simulink library "trw_checksum"  (Simulink 8.2)
settings: Solver=ode1  StartTime=0.0  StopTime=Inf  FixedStep=0.001  RelTol=1e-3
PostLoadFcn:
  | , if any(exist('dsrtsu_mdlpostloadfcn', 'file') == [2, 3, 6]), try dsrtsu_mdlpostloadfcn('Execute', bdroot); catch fprintf('Error in PostLoadFcn (dsrtsu_mdlpostloadfcn) for model "%s":\n %s\n', bdroot, lasterr); end, end,
settings Model: DSRTSU_INTERNAL_RTI_VER=450  DSRTSU_INTERNAL_RTI_TYPE=rti1401  RTICANMMDATA=struct('GeneralSetupData',struct('modelroot','D:\ADAS\ADAS\trunk\ADAS_Softwares\HTDragon\software\sw_development\arch','generalsettings',struct('filesettings',struct('destfolder',struct('Name','RTICANMM_FILES','Check',1),'buildfolder',struct('Name','.','Check',1),'AbsDestfolder',struct('Name','D:\ADAS\ADAS\trunk\ADAS_Softwares\HTDragon\software\sw_development\arch\RTICANMM_FILES'),'AbsBuildfolder',struct('Name','D:\ADAS\ADAS\trunk\ADAS_Softwares\HTDragon\software\sw_development\arch'))),'options',struct('addpaths',1,'rmpaths',1,'addtrcexclusion',logical(1),'cannavigator',struct('checkmonitoring',0),'show_usrtrc',0,'use_usrtrc',0),'advanced',struct('options',[1 1 1 1 1 1 1 1 1 1 1 1 1 1 1 1 1 1 1 1 1 1 1 1 1 1 1 1 1 1 1 1 1 1 1 1 1 1 1 1 1 1 1 1 1 1 1 1 1 1 1 1 1 1 1 1 1 1 1 1 1 1 1 1 1 1 1 1 1 1 1 1 1 1 1 1 1 1 1 1 1 1 1 1 1 1 1 1 1 1 1 1 1 1 1 1 1 1 1 1]),'MPSetup',{{}},'modelname','trw_checksum','block','trw_checksum'))  DSRTSU_INTERNAL_RTIFPGA=40  Creator=11116  LastModifiedBy=11116

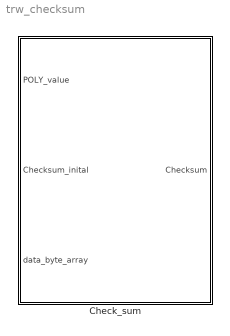
== system trw_checksum ==
  Check_sum : MATLAB Function  TreatAsAtomicUnit=on

== matlab function Check_sum ==
  data: POLY_value input double; Checksum output double; Checksum_inital input double; data_byte_array input double
function Checksum = Check_sum(POLY_value,Checksum_inital,data_byte_array)
Checksum = uint8(Checksum_inital);

    for byte_index = 1 : 1 : 7
        Checksum = bitxor(Checksum,data_byte_array(byte_index));
        
        for bit_index = 0 : 1 : 7
            
            if bitand(Checksum,128)
                Checksum = bitshift(uint8(Checksum),1);
                Checksum = bitxor(Checksum,uint8(POLY_value));
            else
                Checksum = bitshift(uint8(Checksum),1);
            end
            
        end

    end
Checksum = bitcmp(Checksum);
end
